simulink model "ekfeuler"  (R2025b)
settings: Solver=VariableStepAuto  StartTime=0.0  StopTime=10.0  RelTol=1e-3
values from neighbouring files (symbols this model uses):
  dt = u(4)    [ekf_F_jac.m]    (also in ekf_stateprop.m)
undefined symbols (not defined in the file or in its folder): del, WMM2025
libraries: simulink x10, aerolibgravity2 x1
settings Model: Creator=Amal  LastModifiedBy=Amal

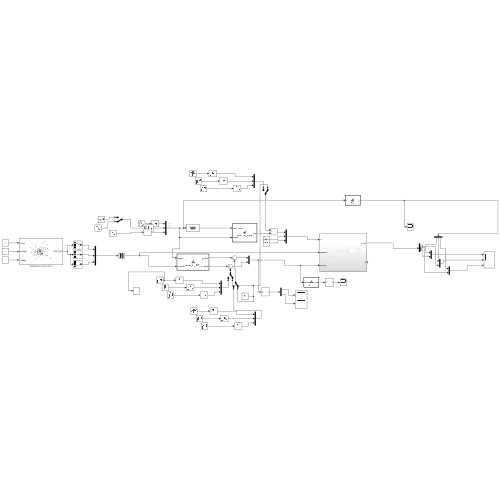
[thumbnail: Simulink's stored preview of the top-level diagram]
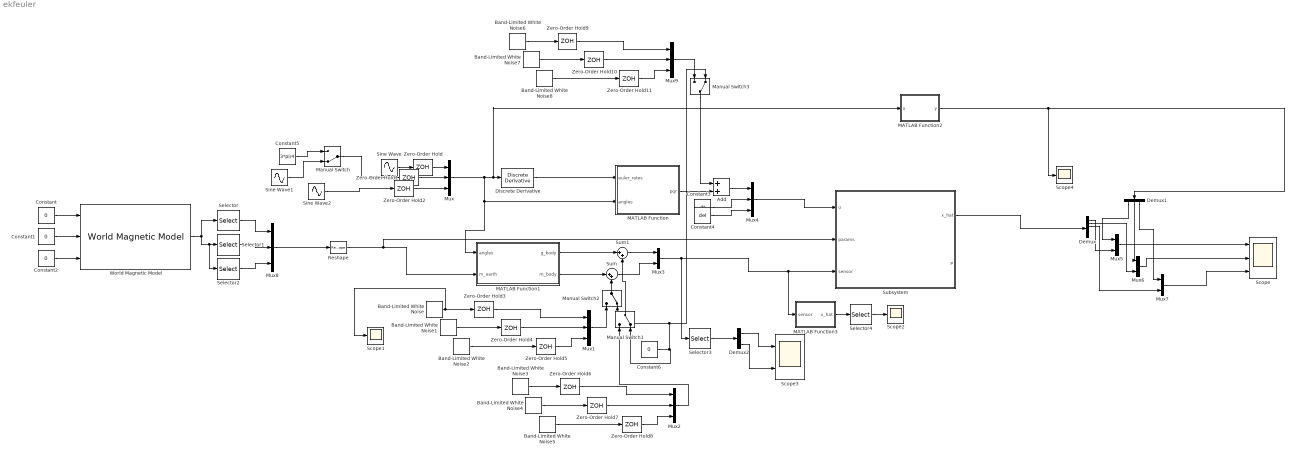
== system ekfeuler ==
  Add : Sum
  Band-Limited White Noise{,1..8} (9 alike) : simulink/Sources/Band-Limited White Noise  Cov=[0.1]*0.1  Ts=dt  seed=[23341]
  Constant{,1..2,6} (4 alike) : Constant  Value=0
  Constant3 : Constant  Value=dt
  Constant4 : Constant  Value=del
  Constant5 : Constant  Value=3*pi/4
  Demux : Demux  Outputs=6
  Demux1 : Demux  Outputs=3
  Demux2 : Demux  Outputs=2
  Discrete Derivative : simulink/Discrete/Discrete Derivative  gainval=1.0  ICPrevScaledInput=[25;50;19]  OutMin=[]  OutMax=[]  OutDataType=fixdt(1, 16)  OutScaling=2^-10  DoSatur=off
  MATLAB Function : MATLAB Function  TreatAsAtomicUnit=on
  MATLAB Function1 : MATLAB Function  TreatAsAtomicUnit=on
  MATLAB Function2 : MATLAB Function  TreatAsAtomicUnit=on
  MATLAB Function3 : MATLAB Function  TreatAsAtomicUnit=on
  Manual Switch{,1..3} (4 alike) : ManualSwitch  CurrentSetting=0
  Mux{,1..2,4,8..9} (6 alike) : Mux  Inputs=3
  Mux{3,5..7} (4 alike) : Mux  Inputs=2
  Reshape : Reshape  OutputDimensionality=Column vector (2-D)
  Scope : Scope  NumInputPorts=3
      settings: ActiveDisplayYMinimum=-3.9269735248205224  ActiveDisplayYMaximum=3.9269765929241758
  Scope1 : Scope
      settings: ActiveDisplayYMinimum=-1  ActiveDisplayYMaximum=1
  Scope2 : Scope
      settings: ActiveDisplayYMinimum=-1.3074518226579008  ActiveDisplayYMaximum=-0.40745141112326932  DataLoggingVariableName=ScopeData2
  Scope3 : Scope  NumInputPorts=2
      settings: ActiveDisplayYMinimum=-8.670884781141984  ActiveDisplayYMaximum=8.6708591802089  DataLoggingVariableName=ScopeData3
  Scope4 : Scope
      settings: ActiveDisplayYMinimum=-3.9269703969658782  ActiveDisplayYMaximum=3.9269863345426019  DataLoggingVariableName=ScopeData4
  Selector : Selector  InputPortWidth=3  IndexOptions=Index vector (dialog)  Indices=[1]  OutputSizes=1
  Selector1 : Selector  InputPortWidth=3  IndexOptions=Index vector (dialog)  Indices=[2]  OutputSizes=1
  Selector2 : Selector  InputPortWidth=3  IndexOptions=Index vector (dialog)  Indices=[3]  OutputSizes=1
  Selector3 : Selector  InputPortWidth=6  IndexOptions=Index vector (dialog)  Indices=[2;3]  OutputSizes=1
  Selector4 : Selector  InputPortWidth=6  IndexOptions=Index vector (dialog)  Indices=[1]  OutputSizes=1
  Sine Wave : Sin  Amplitude=2*pi  SampleTime=0
  Sine Wave1 : Sin  Amplitude=pi  SampleTime=0
  Sine Wave2 : Sin  Amplitude=pi  SampleTime=0
  Subsystem : Subsystem
  Sum : Sum  Inputs=|++
  Sum1 : Sum  Inputs=|++
  World Magnetic Model : aerolibgravity2/World Magnetic Model  model=WMM2025 (2025-2030)  customFile='WMM2025.COF'  units=Metric (MKS)  time_in=off  month=January  day=1  year=2026  action=Error  h_out=off  dec_out=off  inc_out=off  ti_out=off
  Zero-Order Hold{,1..11} (12 alike) : ZeroOrderHold  SampleTime=dt
  wires:
  Sine Wave/1 -> Zero-Order Hold/1
  Sine Wave1/1 -> Manual Switch/2
  Sine Wave2/1 -> Zero-Order Hold2/1
  Discrete Derivative/1 -> MATLAB Function/1(euler_rates)
  Mux/1 -> Discrete Derivative/1, MATLAB Function2/1(u), MATLAB Function/2(angles), MATLAB Function1/1(angles)
  Zero-Order Hold/1 -> Mux/1
  Zero-Order Hold1/1 -> Mux/2
  Zero-Order Hold2/1 -> Mux/3
  Band-Limited White Noise2/1 -> Zero-Order Hold5/1
  Band-Limited White Noise1/1 -> Zero-Order Hold4/1
  Band-Limited White Noise/1 -> Scope1/1, Zero-Order Hold3/1
  Zero-Order Hold3/1 -> Mux1/1
  Zero-Order Hold4/1 -> Mux1/2
  Zero-Order Hold5/1 -> Mux1/3
  Constant2/1 -> World Magnetic Model/3
  Constant1/1 -> World Magnetic Model/2
  Constant/1 -> World Magnetic Model/1
  MATLAB Function1/2(m_body) -> Sum/1
  Band-Limited White Noise3/1 -> Zero-Order Hold6/1
  Band-Limited White Noise5/1 -> Zero-Order Hold8/1
  Band-Limited White Noise4/1 -> Zero-Order Hold7/1
  Zero-Order Hold7/1 -> Mux2/2
  Zero-Order Hold6/1 -> Mux2/1
  Zero-Order Hold8/1 -> Mux2/3
  MATLAB Function1/1(g_body) -> Sum1/1
  Sum1/1 -> Mux3/1
  Sum/1 -> Mux3/2
  Constant3/1 -> Mux4/2
  Constant4/1 -> Mux4/3
  Demux1/1 -> Mux5/1
  Demux/1 -> Mux5/2
  Demux1/2 -> Mux6/1
  Demux/2 -> Mux6/2
  Demux/3 -> Mux7/2
  Demux1/3 -> Mux7/1
  Mux5/1 -> Scope/1
  Mux6/1 -> Scope/2
  Mux7/1 -> Scope/3
  Selector/1 -> Mux8/1
  Selector1/1 -> Mux8/2
  Selector2/1 -> Mux8/3
  Reshape/1 -> Subsystem/2(params), MATLAB Function1/2(m_earth)
  World Magnetic Model/1 -> Selector2/1, Selector1/1, Selector/1
  Mux8/1 -> Reshape/1
  Subsystem/1(x_hat) -> Demux/1
  MATLAB Function2/1(y) -> Scope4/1, Demux1/1
  Zero-Order Hold11/1 -> Mux9/3
  Zero-Order Hold9/1 -> Mux9/1
  Zero-Order Hold10/1 -> Mux9/2
  Band-Limited White Noise6/1 -> Zero-Order Hold9/1
  Band-Limited White Noise8/1 -> Zero-Order Hold11/1
  Band-Limited White Noise7/1 -> Zero-Order Hold10/1
  Add/1 -> Mux4/1
  MATLAB Function/1(pqr) -> Add/2
  Mux4/1 -> Subsystem/1(u)
  MATLAB Function3/1(x_hat) -> Selector4/1
  Mux3/1 -> Selector3/1, MATLAB Function3/1(sensor), Subsystem/3(sensor)
  Selector3/1 -> Demux2/1
  Demux2/1 -> Scope3/1
  Demux2/2 -> Scope3/2
  Constant5/1 -> Manual Switch/1
  Manual Switch/1 -> Zero-Order Hold1/1
  Constant6/1 -> Manual Switch1/2, Manual Switch2/2, Manual Switch3/2
  Mux2/1 -> Manual Switch1/1
  Manual Switch2/1 -> Sum/2
  Manual Switch1/1 -> Sum1/2
  Mux1/1 -> Manual Switch2/1
  Mux9/1 -> Manual Switch3/1
  Manual Switch3/1 -> Add/1
  Selector4/1 -> Scope2/1

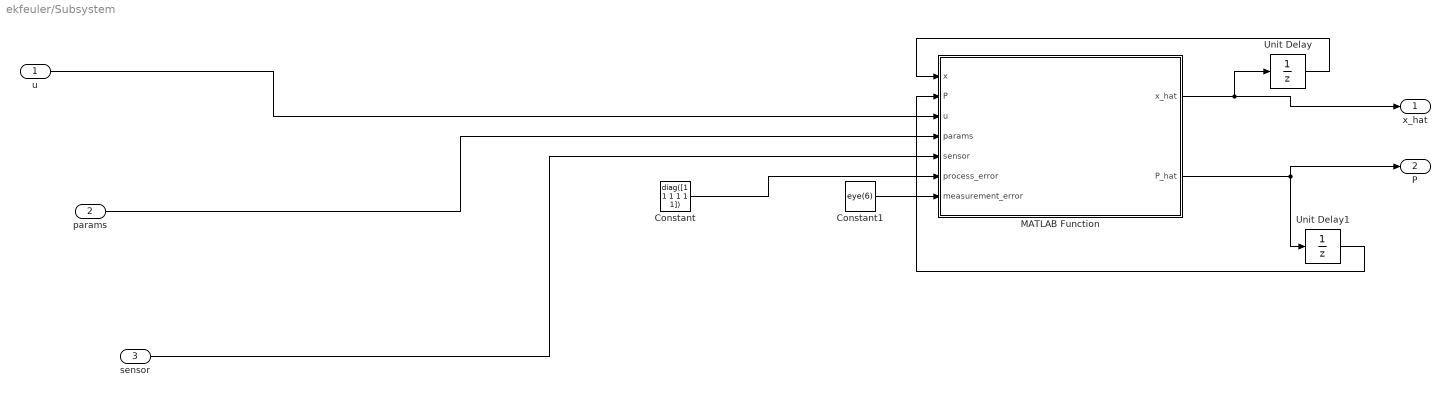
== system ekfeuler/Subsystem ==
  u : Inport
  params : Inport  Port=2
  sensor : Inport  Port=3
  Constant : Constant  Value=diag([1 1 1 1 1 1])
  Constant1 : Constant  Value=eye(6)
  MATLAB Function : MATLAB Function  TreatAsAtomicUnit=on
  Unit Delay : UnitDelay  InitialCondition=[pi/4;0;0;0;0;0]  SampleTime=dt  HasFrameUpgradeWarning=on
  Unit Delay1 : UnitDelay  InitialCondition=diag([1 1 1 1 1 1]);  SampleTime=dt  HasFrameUpgradeWarning=on
  x_hat : Outport
  P : Outport  Port=2
  wires:
  Constant/1 -> MATLAB Function/6(process_error)
  Constant1/1 -> MATLAB Function/7(measurement_error)
  params/1 -> MATLAB Function/4(params)
  u/1 -> MATLAB Function/3(u)
  sensor/1 -> MATLAB Function/5(sensor)
  MATLAB Function/1(x_hat) -> Unit Delay/1, x_hat/1
  MATLAB Function/2(P_hat) -> Unit Delay1/1, P/1
  Unit Delay/1 -> MATLAB Function/1(x)
  Unit Delay1/1 -> MATLAB Function/2(P)

== matlab function ekfeuler/MATLAB Function1 ==
  data: angles input; g_body output; m_earth input; m_body output
function [g_body,m_body] = euler_to_RIB(angles,m_earth)
    % angles : [phi; theta; psi] in radians
    
    phi   = angles(1);
    theta = angles(2);
    psi   = angles(3);


    % Pre-calculate trig terms
    sr = sin(phi);   cr = cos(phi);
    sp = sin(theta); cp = cos(theta);
    sy = sin(psi);   cy = cos(psi);

    if abs(cp) <1e-6
        cp = 1e-6;
    end
        
    % Rotation Matrix: Inertial to Body
    RIB = [ cp*cy,                cp*sy,               -sp;
             sr*sp*cy - cr*sy,     sr*sp*sy + cr*cy,     sr*cp;
             cr*sp*cy + sr*sy,     cr*sp*sy - sr*cy,     cr*cp ];

    g_body = RIB* [0;0;9.81];
    m_body = RIB* m_earth;
end

== matlab function ekfeuler/MATLAB Function ==
  data: euler_rates input; pqr output; angles input
function pqr = euler_to_body(euler_rates, angles)
    % euler_rates : [phi_dot; theta_dot; psi_dot]
    % angles      : [phi; theta; psi]

    phi   = angles(1);
    theta = angles(2);
    % psi is not required for this transformation

    phid   = euler_rates(1);
    thetad = euler_rates(2);
    psid   = euler_rates(3);

    % Pre-calculate trig terms
    sr = sin(phi);   cr = cos(phi);
    sp = sin(theta); cp = cos(theta);

    % Transformation Matrix (Euler rates to Body rates)
    % p = phid - psid * sin(theta)
    % q = thetad * cos(phi) + psid * sin(phi) * cos(theta)
    % r = -thetad * sin(phi) + psid * cos(phi) * cos(theta)
    
    M = [ 1,  0,   -sp;
          0,  cr,  sr*cp;
          0, -sr,  cr*cp ];

    pqr = M * [phid; thetad; psid];
end

== matlab function ekfeuler/MATLAB Function2 ==
  data: u input; y output
function y = fcn(u)
y = atan2(sin(u),cos(u));
if abs(u(2))>= pi/2
    u(1)= u(1) + pi;
    u(2) = pi - u(2);
    u(3) = u(3) + pi;
    y = atan2(sin(u),cos(u));
end

end

== matlab function ekfeuler/MATLAB Function3 ==
  data: sensor input; x_hat output
function x_hat = fcn(sensor)

 gx = sensor(1); gy = sensor(2); gz = sensor(3);
        mx = sensor(4); my = sensor(5); mz = sensor(6);
        x_hat = zeros(6,1);
       % Accelerometer-based Roll and Pitch
r = atan2(gy, gz);
p = atan2(-gx, sqrt(gy^2 + gz^2));

% Magnetometer-based Yaw (Tilt-Compensated)
% Note the specific grouping of terms in the denominator
mx_h = mx*cos(p) + my*sin(r)*sin(p) + mz*cos(r)*sin(p);
my_h = my*cos(r) - mz*sin(r);

y = atan2(-my_h, mx_h);

% Assign to x_hat
x_hat(1) = r;
x_hat(2) = p;
x_hat(3) = y;
end

== matlab function ekfeuler/Subsystem/MATLAB Function ==
  data: x input; P input; u input; x_hat output; params input; sensor input; P_hat output; process_error input; measurement_error input
function [x_hat, P_hat] = ekf(x,P, u, params,sensor, process_error, measurement_error)
    phi = x(1); theta = x(2); psi = x(3);  del = u(5);

    if (pi/2 - abs(theta)) <= del
        gx = sensor(1); gy = sensor(2); gz = sensor(3);
        mx = sensor(4); my = sensor(5); mz = sensor(6);
        x_hat = zeros(6,1);
       % Accelerometer-based Roll and Pitch
r = atan2(gy, gz);
p = atan2(-gx, sqrt(gy^2 + gz^2));

% Magnetometer-based Yaw (Tilt-Compensated)
% Note the specific grouping of terms in the denominator
mx_h = mx*cos(p) + my*sin(r)*sin(p) + mz*cos(r)*sin(p);
my_h = my*cos(r) - mz*sin(r);

y = atan2(-my_h, mx_h);

% Assign to x_hat
x_hat(1) = r;
x_hat(2) = p;
x_hat(3) = y;
        P_hat = P;
    else
    Q = process_error;
    R = measurement_error;

    pqr = u(1:3); 
    bias = x(4:6);
    p = u(1); q = u(2); r = u(3);
    dt = u(4);

    g = 9.81;
    g_I = [0; 0; g];

    mI = params(1:3);

    mN = mI(1); mE = mI(2); mD = mI(3);



   % Pre-calculate trig terms for efficiency
    sr = sin(phi);   cr = cos(phi);
    sp = sin(theta); cp = cos(theta);
    tp = tan(theta);      % tan(theta)
    sy = sin(psi);   cy = cos(psi);
    cp2 = cp^2;      % cos^2(theta)

    % Transformation matrix
    T          = [ 1, sr*tp, cr*tp; 
                   0, cr,    -sr; 
                   0, sr/cp, cr/cp ];
    T_final = [T, zeros(3);zeros(3),zeros(3)];

    x_dot = T_final * [pqr-bias;0;0;0];
    x_next = x + x_dot * dt;
    
    % Wrap angles to [-pi, pi]
    for i = 1:3
     x_next(i) = atan2(sin(x_next(i)), cos(x_next(i))); 
    end

 % Prevent singularity at pitch = +/- 90 degrees
     if (pi/2 - abs(x_next(2)))< del
        % x_next(2) = sign(x_next(2)) * (pi/2 - delta);

     
        gx = sensor(1); gy = sensor(2); gz = sensor(3);
        mx = sensor(4); my = sensor(5); mz = sensor(6);
        x_hat = zeros(6,1);
       % Accelerometer-based Roll and Pitch
r = atan2(gy, gz);
p = atan2(-gx, sqrt(gy^2 + gz^2));

% Magnetometer-based Yaw (Tilt-Compensated)
% Note the specific grouping of terms in the denominator
mx_h = mx*cos(p) + my*sin(r)*sin(p) + mz*cos(r)*sin(p);
my_h = my*cos(r) - mz*sin(r);

y = atan2(-my_h, mx_h);

% Assign to x_hat
x_hat(1) = r;
x_hat(2) = p;
x_hat(3) = y;
        P_hat = P;
   else
    
    
    bp = bias(1); bq = bias(2); br = bias(3);

    % Continuous-time Jacobian (df/dx)
    dfdx = zeros(6,6);

    % Row 1: d(phi_dot)/dx
    dfdx(1,1) = (q-bq)*cr*tp - (r-br)*sr*tp;         
    dfdx(2,1) = -(q-bq)*sr - (r-br)*cr;              
    dfdx(3,1) = ((q-bq)*cr - (r-br)*sr) / cp;        

    dfdx(1,2) = ((q-bq)*sr + (r-br)*cr) / cp2;       
    dfdx(2,2) = 0;                          
    dfdx(3,2) = ((q-bq)*sr + (r-br)*cr) * sp / cp2;   

    
   
    
    dfdx(1,3) = 0;   
    dfdx(2,3) = 0;                        
    dfdx(3,3) = 0;       

    dfdx(1,4) = -1;   
    dfdx(2,4) = 0;                        
    dfdx(3,4) = 0;  

    dfdx(1,5) = -sr*tp;   
    dfdx(2,5) = -cr;                        
    dfdx(3,5) = -sr/cp;  

    dfdx(1,6) = -cr*tp;   
    dfdx(2,6) = sr;                        
    dfdx(3,6) = -cr/cp; 


 
    % Discrete-time Jacobian: F = I + df/dx * dt
    F = eye(6) + dfdx * dt;
    
   
    P_next = F*P*(F') + Q;
    
     phi = x_next(1); theta = x_next(2); psi = x_next(3);
    
    
     % Pre-calculate trig
    sr = sin(phi);   cr = cos(phi);
    sp = sin(theta); cp = cos(theta);
    sy = sin(psi);   cy = cos(psi);

    % Rotation Matrix: Inertial to Body (R_x * R_y * R_z)
    R_IB = [ cp*cy,                cp*sy,               -sp;
             sr*sp*cy - cr*sy,     sr*sp*sy + cr*cy,     sr*cp;
             cr*sp*cy + sr*sy,     cr*sp*sy - sr*cy,     cr*cp ];

    % Predicted measurements
    h_acc = R_IB * g_I;
    h_mag = R_IB * params;

    % Combine into a single 6x1 measurement vector
    h = [h_acc; h_mag];



    H = zeros(6,6);

    %% Column 1 
   
    H(1,1) = 0;
    H(2,1) = cr*cp*g;
    H(3,1) = -sr*cp*g;
    H(4,1) = 0;
    H(5,1) = (cr*sp*cy + sr*sy)*mN + (cr*sp*sy - sr*cy)*mE + cr*cp*mD;
    H(6,1) = (-sr*sp*cy + cr*sy)*mN + (-sr*sp*sy - cr*cy)*mE - sr*cp*mD;

  %% Column 2
    H(1,2) =  -cp*g;
    H(2,2) =  -sr*sp*g;
    H(3,2) =  -cr*sp*g;
     
    H(4,2) = -sp*cy*mN - sp*sy*mE - cp*mD;
    H(5,2) = sr*cp*cy*mN + sr*cp*sy*mE - sr*sp*mD;
    H(6,2) = cr*cp*cy*mN + cr*cp*sy*mE - cr*sp*mD;
   

   

   %% Column 3
    H(1,3) = 0;
    H(2,3) = 0;
    H(3,3) = 0;
    H(4,3) = -cp*sy*mN + cp*cy*mE;
    H(5,3) = (-sr*sp*sy - cr*cy)*mN + (sr*sp*cy - cr*sy)*mE;
    H(6,3) = (-cr*sp*sy + sr*cy)*mN + (cr*sp*cy + sr*sy)*mE;

    %Column 4,5,6 all are zero due to mathematically no relation between
    %differentiating variable and the h matrix (bp,bq,br)

      K = P_next*(H')/(H*P_next*H'+R);

      innovation = sensor - h;
     
      x_hat = x_next + K*(innovation);
    
    for i = 1:3
      x_hat(i) = atan2(sin(x_hat(i)), cos(x_hat(i))); 
    end
        
       % Prevent singularity at pitch = +/- 90 degrees
     if abs(x_hat(2)) >= pi/2
         x_hat(2) = sign(x_hat(2) * (pi/2 - del));
     end

      P_hat = (eye(6)- K*H)*P_next;
     end
    end
    if abs(x_hat(2)) >= pi/2 
        x_hat(1)= x_hat(1) + pi;
        x_hat(2)= pi - x_hat(2);
        x_hat(3)= x_hat(3) + pi;
         % Wrap angles to [-pi, pi]
    for i = 1:3
     x_hat(i) = atan2(sin(x_hat(i)), cos(x_hat(i))); 
    end
    end

end
